simulink model "Subsystem1"  (R2020a)
settings: Solver=FixedStepAuto  StartTime=0.0  StopTime=20  FixedStep=1  RelTol=1e-3
settings Model: Creator=NIKITA  LastModifiedBy=NIKITA
settings DataIOCC: SaveOutput=off  SaveTime=off

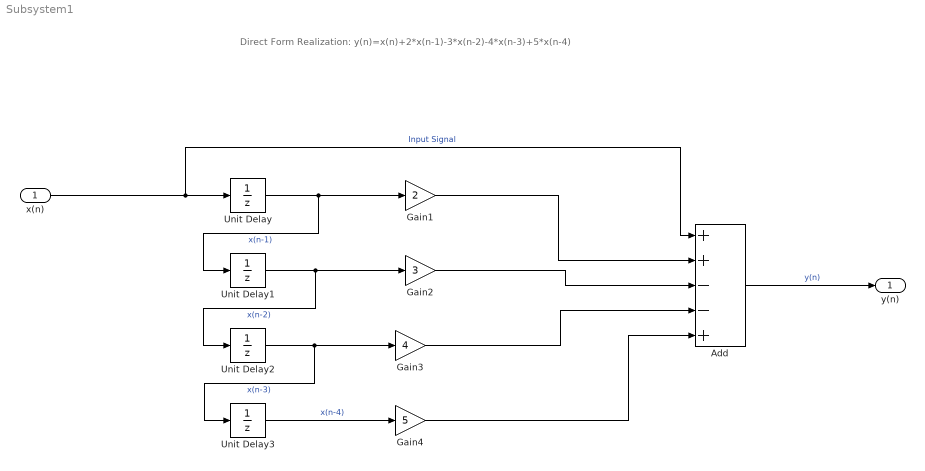
== system Subsystem1 ==
  note: Direct Form Realization:
      | y(n)=x(n)+2*x(n-1)-3*x(n-2)-4*x(n-3)+5*x(n-4)
  x(n) : Inport  OutDataTypeStr=double  PortDimensions=[1 1]  SampleTime=[1,0]
  Add : Sum  Inputs=++--+
  Gain1 : Gain  Gain=2
  Gain2 : Gain  Gain=3
  Gain3 : Gain  Gain=4
  Gain4 : Gain  Gain=5
  Unit Delay{,1..3} (4 alike) : UnitDelay  SampleTime=-1  HasFrameUpgradeWarning=on
  y(n) : Outport  OutDataTypeStr=double  PortDimensions=[1 1]  SampleTime=[1,0]
  wires:
  Gain1/1 -> Add/2
  Unit Delay/1 -> Gain1/1, Unit Delay1/1  "x(n-1)"
  Gain2/1 -> Add/3
  Gain3/1 -> Add/4
  Unit Delay1/1 -> Unit Delay2/1, Gain2/1  "x(n-2)"
  Unit Delay3/1 -> Gain4/1  "x(n-4)"
  Add/1 -> y(n)/1  "y(n)"
  x(n)/1 -> Add/1, Unit Delay/1  "Input Signal"
  Unit Delay2/1 -> Unit Delay3/1, Gain3/1  "x(n-3)"
  Gain4/1 -> Add/5
